simulink model "Rob_Diff_Erno_1R1"  (R2013a)
settings: Solver=ode45  StartTime=0.0  StopTime=inf  RelTol=1e-3
undefined symbols (not defined in the file): Corp1, RoataMare1, Rob_Diff_Erno_1, RootPart
libraries: mblibv1 x17
settings Model: Creator=Claudiu  LastModifiedBy=Claudiu
settings SimMechanicsCC: VisOnUpdateDiagram=on  VisDuringSimulation=on

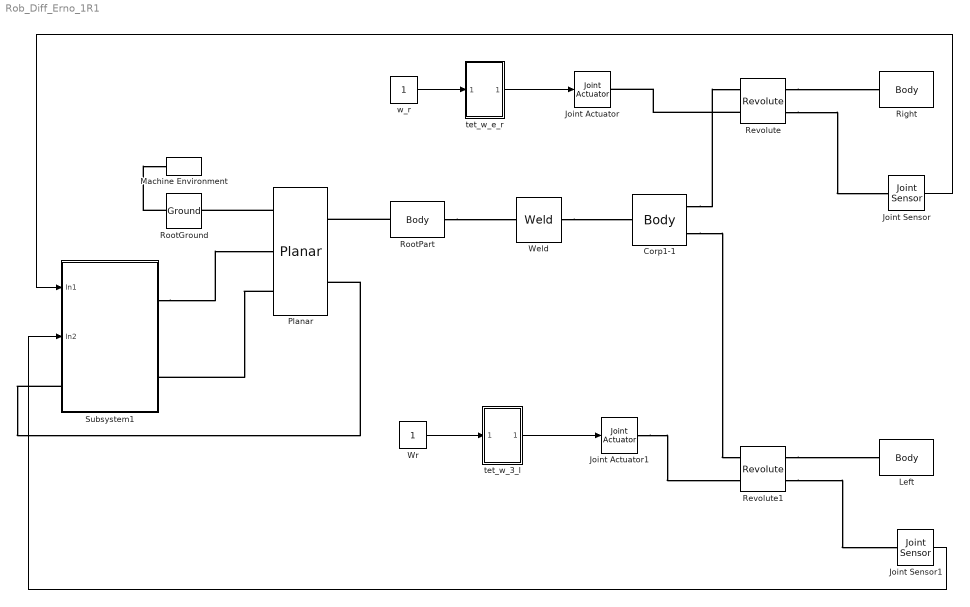
== system Rob_Diff_Erno_1R1 ==
  Corp1-1 : mblibv1/Bodies/Body  LConnTagsString=CS2  RConnTagsString=CS3|CS4  UpdateFromCAD=on  PMImportedID=Corp1-1  DialogClass=MechanicalBodyBlock  Mass=50.6599  MassUnits=kg  InertiaUnits=kg*m^2  Inertia=[1.29318,-0.000149252,5.94621e-08;-0.000149252,0.603177,0.00116217;5.94621e-08,0.00116217,1.81376]  Shape=Cylinder  ShapeDims=[1 1]  ShapeUnits=m  ShapeUse=false  Density=1  DensityUnits=kg/m^3  DensityUse=false  GraphicsMode=GFXFILE  GraphicsFileName=Rob_Diff_Erno_1 - Corp1-1.STL  BodyColorSelMode=COLORPALETTE  BodyColor=[0.894118;0.913725;0.929412]  AttachedToCS=CS1  CG=Right$CG$[-3.54762e-11 0.213212 0.000124454]$WORLD$WORLD$m$[1 0 0;0 1 0;0 0 1]$3x3 Transform$rad$WORLD$false$Corp1-1::CG(AUTOGEN)  WorkingFrames=Right$CS1$[0 0 0]$WORLD$WORLD$m$[1 0 0;0 1 0;0 0 1]$3x3 Transform$rad$WORLD$false$Corp1-1::CS1(AUTOGEN)#Left$CS2$[-3.54762e-11 0.213212 0.000124454]$WORLD$WORLD$m$[1 0 0;0 1 0;0 0 1]$3x3 Transform$rad$WORLD$true$Corp1-1:-:Rob_Diff_Erno_1/RootPart::Corp1-1(AUTOGEN)#Right$CS3$[-0.27 0.253869 0]$WORLD$WORLD$m$[1 0 0;0 1 0;0 0 1]$3x3 Transform$rad$WORLD$true$Corp1-1:-:RoataMare1-1::Corp1-1(AUTOGEN)#Right$CS4$[0.27 0.254678 0]$WORLD$WORLD$m$[1 0 0;0 1 0;0 0 1]$3x3 Transform$rad$WORLD$true$Corp1-1:-:RoataMare1-2::Corp1-1(AUTOGEN)  CGPos=[-3.54762e-11 0.213212 0.000124454]  CGRot=[1 0 0;0 1 0;0 0 1]  CS0Pos=[]  CS0Rot=[]  CS1Pos=[0 0 0]  CS1Rot=[1 0 0;0 1 0;0 0 1]  CS2Pos=[-3.54762e-11 0.213212 0.000124454]  CS2Rot=[1 0 0;0 1 0;0 0 1]  CS3Pos=[-0.27 0.253869 0]  CS3Rot=[1 0 0;0 1 0;0 0 1]  CS4Pos=[0.27 0.254678 0]  CS4Rot=[1 0 0;0 1 0;0 0 1]  CS5Pos=[]  CS5Rot=[]  CS6Pos=[]  CS6Rot=[]  CS7Pos=[]  CS7Rot=[]  CS8Pos=[]  CS8Rot=[]  CS9Pos=[]  CS9Rot=[]  CS10Pos=[]  CS10Rot=[]  CS11Pos=[]  CS11Rot=[]  CS12Pos=[]  CS12Rot=[]  CS13Pos=[]  CS13Rot=[]  CS14Pos=[]  CS14Rot=[]  CS15Pos=[]  CS15Rot=[]  CS16Pos=[]  CS16Rot=[]  CS17Pos=[]  CS17Rot=[]  CS18Pos=[]  CS18Rot=[]  CS19Pos=[]  CS19Rot=[]  CS20Pos=[]  CS20Rot=[]
  Joint Actuator : mblibv1/Sensors &  Actuators/Joint Actuator  UpdateFromCAD=off  PhysicalDomain=Mechanical  PortType=blob  ActuationStyle=Motion  AngleUnits=deg  ArcVelocityUnits=deg/s  ArcAccelerationUnits=deg/s^2  CoordPositionUnits=m  VelocityUnits=m/s  AccelerationUnits=m/s^2  ForceUnits=N  TorqueUnits=N*m  ActiveIO=on  Width=3  DialogClass=MechanicalActuatorBlock  Primitive=R1  ReferenceFrame=Absolute (World)
  Joint Actuator1 : mblibv1/Sensors &  Actuators/Joint Actuator  UpdateFromCAD=off  PhysicalDomain=Mechanical  PortType=blob  ActuationStyle=Motion  AngleUnits=deg  ArcVelocityUnits=deg/s  ArcAccelerationUnits=deg/s^2  CoordPositionUnits=m  VelocityUnits=m/s  AccelerationUnits=m/s^2  ForceUnits=N  TorqueUnits=N*m  ActiveIO=on  Width=3  DialogClass=MechanicalActuatorBlock  Primitive=R1  ReferenceFrame=Absolute (World)
  Joint Sensor : mblibv1/Sensors &  Actuators/Joint Sensor  UpdateFromCAD=off  PhysicalDomain=Mechanical  PortType=blob  Muxed=on  Pose=off  Angle=off  AngleUnits=rad  ArcVelocity=on  ArcVelocityUnits=rad/s  ArcAcceleration=off  ArcAccelerationUnits=deg/s^2  CoordPosition=on  CoordPositionUnits=m  Velocity=off  VelocityUnits=m/s  Acceleration=off  AccelerationUnits=m/s^2  Quaternion=on  QuaternionDT=off  QuaternionDDT=off  QuaternionUnits=off  OutputVector=[1]  ActiveIO=on  Width=1  DialogClass=MechanicalSensorBlock  Primitive=R1  Force=off  ForceUnits=N  Torque=off  TorqueUnits=N*m  ReferenceFrame=Absolute (World)  ReactionSensedSide=Base  ReactionReferenceFrame=Absolute (World)  ReactionForce=off  ReactionForceUnits=N  ReactionMoment=off  ReactionMomentUnits=N*m
  Joint Sensor1 : mblibv1/Sensors &  Actuators/Joint Sensor  UpdateFromCAD=off  PhysicalDomain=Mechanical  PortType=blob  Muxed=on  Pose=off  Angle=off  AngleUnits=rad  ArcVelocity=on  ArcVelocityUnits=rad/s  ArcAcceleration=off  ArcAccelerationUnits=deg/s^2  CoordPosition=on  CoordPositionUnits=m  Velocity=off  VelocityUnits=m/s  Acceleration=off  AccelerationUnits=m/s^2  Quaternion=on  QuaternionDT=off  QuaternionDDT=off  QuaternionUnits=off  OutputVector=[1]  ActiveIO=on  Width=1  DialogClass=MechanicalSensorBlock  Primitive=R1  Force=off  ForceUnits=N  Torque=off  TorqueUnits=N*m  ReferenceFrame=Absolute (World)  ReactionSensedSide=Base  ReactionReferenceFrame=Absolute (World)  ReactionForce=off  ReactionForceUnits=N  ReactionMoment=off  ReactionMomentUnits=N*m
  Left : mblibv1/Bodies/Body  LConnTagsString=CS2  UpdateFromCAD=on  PMImportedID=RoataMare1-2  DialogClass=MechanicalBodyBlock  Mass=3.13776  MassUnits=kg  InertiaUnits=kg*m^2  Inertia=[0.016344,3.64267e-07,-4.71483e-11;3.64267e-07,0.0163435,-1.65655e-11;-4.71483e-11,-1.65655e-11,0.0280968]  Shape=Cylinder  ShapeDims=[1 1]  ShapeUnits=m  ShapeUse=false  Density=1  DensityUnits=kg/m^3  DensityUse=false  GraphicsMode=GFXFILE  GraphicsFileName=Rob_Diff_Erno_1 - RoataMare1-2.STL  BodyColorSelMode=COLORPALETTE  BodyColor=[0.792157;0.819608;0.933333]  AttachedToCS=CS1  CG=Right$CG$[0.22 0.254684 2.07949e-06]$WORLD$WORLD$m$[0 0 -1;0.683357 0.730084 0;0.730084 -0.683357 0]$3x3 Transform$rad$WORLD$false$RoataMare1-2::CG(AUTOGEN)  WorkingFrames=Right$CS1$[0.22 0.254678 0]$WORLD$WORLD$m$[0 0 -1;0.683357 0.730084 0;0.730084 -0.683357 0]$3x3 Transform$rad$WORLD$false$RoataMare1-2::CS1(AUTOGEN)#Left$CS2$[0.27 0.254678 0]$WORLD$WORLD$m$[1 0 0;0 1 0;0 0 1]$3x3 Transform$rad$WORLD$true$Corp1-1:-:RoataMare1-2::RoataMare1-2(AUTOGEN)  CGPos=[0.22 0.254684 2.07949e-06]  CGRot=[0 0 -1;0.683357 0.730084 0;0.730084 -0.683357 0]  CS0Pos=[]  CS0Rot=[]  CS1Pos=[0.22 0.254678 0]  CS1Rot=[0 0 -1;0.683357 0.730084 0;0.730084 -0.683357 0]  CS2Pos=[0.27 0.254678 0]  CS2Rot=[1 0 0;0 1 0;0 0 1]  CS3Pos=[]  CS3Rot=[]  CS4Pos=[]  CS4Rot=[]  CS5Pos=[]  CS5Rot=[]  CS6Pos=[]  CS6Rot=[]  CS7Pos=[]  CS7Rot=[]  CS8Pos=[]  CS8Rot=[]  CS9Pos=[]  CS9Rot=[]  CS10Pos=[]  CS10Rot=[]  CS11Pos=[]  CS11Rot=[]  CS12Pos=[]  CS12Rot=[]  CS13Pos=[]  CS13Rot=[]  CS14Pos=[]  CS14Rot=[]  CS15Pos=[]  CS15Rot=[]  CS16Pos=[]  CS16Rot=[]  CS17Pos=[]  CS17Rot=[]  CS18Pos=[]  CS18Rot=[]  CS19Pos=[]  CS19Rot=[]  CS20Pos=[]  CS20Rot=[]
  Machine Environment : mblibv1/Bodies/Machine Environment  PortType=env  PhysicalDomain=Mechanical  DialogTemplateClass=MECH.MachineEnvironment  SyncWhenCopied=off  Gravity=[0 0 0]  GravityUnits=m/s^2  GravityAsSignal=off  Dimensionality=Auto-detect  AnalysisType=Forward dynamics  LinearAssemblyTolerance=1e-3  LinearAssemblyToleranceUnits=m  AngularAssemblyTolerance=1e-3  AngularAssemblyToleranceUnits=rad  ConstraintSolverType=Stabilizing  ConstraintRelTolerance=1e-4  ConstraintAbsTolerance=1e-4  UseRobustSingularityHandling=off  RedundancyAnalysisToleranceType=Automatically select tolerance  RedundancyAnalysisTolerance=1e-14  StatePerturbationType=Fixed  PerturbationSize=1e-5  VisualizeMachine=on  BodyVisualizationType=Use model default body geometries  BodyColorSelMode=Use model default  DefaultBodyColor=[1 0 0]
  Planar : mblibv1/Joints/Planar  LConnTagsString=__newl0|SA1|SA2  RConnTagsString=__newr0|SA1  UpdateFromCAD=off  NumSAPorts=3  CutJoint=off  MarkAsCut=off  Primitives=prismatic_prismatic  PrimitiveProps=P1$World$[1 0 0]$prismatic#P2$World$[0 1 0]$prismatic#R1$World$[0 0 1]$revolute  DialogClass=JointBlock  P1Axis=[1 0 0]  P2Axis=[0 1 0]  R1Axis=[0 0 1]
  Revolute : mblibv1/Joints/Revolute  LConnTagsString=__newl0|SA1  RConnTagsString=__newr0|SA1  UpdateFromCAD=on  PMImportedID=Corp1-1:-:RoataMare1-1  NumSAPorts=2  CutJoint=off  MarkAsCut=off  Primitives=prismatic  PrimitiveProps=R1$World$[1,0,0]$revolute  DialogClass=JointBlock  R1Axis=[1,0,0]
  Revolute1 : mblibv1/Joints/Revolute  LConnTagsString=__newl0|SA1  RConnTagsString=__newr0|SA1  UpdateFromCAD=on  PMImportedID=Corp1-1:-:RoataMare1-2  NumSAPorts=2  CutJoint=off  MarkAsCut=off  Primitives=prismatic  PrimitiveProps=R1$World$[-1,0,0]$revolute  DialogClass=JointBlock  R1Axis=[-1,0,0]
  Right : mblibv1/Bodies/Body  LConnTagsString=CS2  UpdateFromCAD=on  PMImportedID=RoataMare1-1  DialogClass=MechanicalBodyBlock  Mass=3.13776  MassUnits=kg  InertiaUnits=kg*m^2  Inertia=[0.016344,3.64267e-07,-4.71483e-11;3.64267e-07,0.0163435,-1.65655e-11;-4.71483e-11,-1.65655e-11,0.0280968]  Shape=Cylinder  ShapeDims=[1 1]  ShapeUnits=m  ShapeUse=false  Density=1  DensityUnits=kg/m^3  DensityUse=false  GraphicsMode=GFXFILE  GraphicsFileName=Rob_Diff_Erno_1 - RoataMare1-1.STL  BodyColorSelMode=COLORPALETTE  BodyColor=[0.792157;0.819608;0.933333]  AttachedToCS=CS1  CG=Right$CG$[-0.22 0.253871 -6.67283e-06]$WORLD$WORLD$m$[0 0 1;-0.325894 0.945406 0;-0.945406 -0.325894 0]$3x3 Transform$rad$WORLD$false$RoataMare1-1::CG(AUTOGEN)  WorkingFrames=Right$CS1$[-0.22 0.253869 0]$WORLD$WORLD$m$[0 0 1;-0.325894 0.945406 0;-0.945406 -0.325894 0]$3x3 Transform$rad$WORLD$false$RoataMare1-1::CS1(AUTOGEN)#Left$CS2$[-0.27 0.253869 0]$WORLD$WORLD$m$[1 0 0;0 1 0;0 0 1]$3x3 Transform$rad$WORLD$true$Corp1-1:-:RoataMare1-1::RoataMare1-1(AUTOGEN)  CGPos=[-0.22 0.253871 -6.67283e-06]  CGRot=[0 0 1;-0.325894 0.945406 0;-0.945406 -0.325894 0]  CS0Pos=[]  CS0Rot=[]  CS1Pos=[-0.22 0.253869 0]  CS1Rot=[0 0 1;-0.325894 0.945406 0;-0.945406 -0.325894 0]  CS2Pos=[-0.27 0.253869 0]  CS2Rot=[1 0 0;0 1 0;0 0 1]  CS3Pos=[]  CS3Rot=[]  CS4Pos=[]  CS4Rot=[]  CS5Pos=[]  CS5Rot=[]  CS6Pos=[]  CS6Rot=[]  CS7Pos=[]  CS7Rot=[]  CS8Pos=[]  CS8Rot=[]  CS9Pos=[]  CS9Rot=[]  CS10Pos=[]  CS10Rot=[]  CS11Pos=[]  CS11Rot=[]  CS12Pos=[]  CS12Rot=[]  CS13Pos=[]  CS13Rot=[]  CS14Pos=[]  CS14Rot=[]  CS15Pos=[]  CS15Rot=[]  CS16Pos=[]  CS16Rot=[]  CS17Pos=[]  CS17Rot=[]  CS18Pos=[]  CS18Rot=[]  CS19Pos=[]  CS19Rot=[]  CS20Pos=[]  CS20Rot=[]
  RootGround : mblibv1/Bodies/Ground  UpdateFromCAD=on  PMImportedID=RootGround  LeftPortType=env  RightPortType=workingframe  PhysicalDomain=Mechanical  DialogClass=GroundBlock  CoordPosition=[-3.1566e-11,0.217738,0.000110483]  CoordPositionUnits=m  StateVectorMgrId=0  MachineId=[1 0]  ShowEnvPort=on
  RootPart : mblibv1/Bodies/Body  LConnTagsString=CS3  RConnTagsString=CS2  UpdateFromCAD=on  PMImportedID=Rob_Diff_Erno_1/RootPart  DialogClass=MechanicalBodyBlock  Mass=0  MassUnits=kg  InertiaUnits=kg*m^2  Inertia=[0,0,0;0,0,0;0,0,0]  Shape=Cylinder  ShapeDims=[1 1]  ShapeUnits=m  ShapeUse=false  Density=1  DensityUnits=kg/m^3  DensityUse=false  GraphicsMode=MACHINE_DEFAULT  BodyColorSelMode=MACHINE_DEFAULT  BodyColor=[1;0;0]  AttachedToCS=CS1  CG=Right$CG$[-3.1566e-11 0.217738 0.000110483]$WORLD$WORLD$m$[1 0 0;0 1 0;0 0 1]$3x3 Transform$rad$WORLD$false$Rob_Diff_Erno_1/RootPart::CG(AUTOGEN)  WorkingFrames=Right$CS1$[0 0 0]$WORLD$WORLD$m$[1 0 0;0 1 0;0 0 1]$3x3 Transform$rad$WORLD$false$Rob_Diff_Erno_1/RootPart::CS1(AUTOGEN)#Right$CS2$[-3.54762e-11 0.213212 0.000124454]$WORLD$WORLD$m$[1 0 0;0 1 0;0 0 1]$3x3 Transform$rad$WORLD$true$Corp1-1:-:Rob_Diff_Erno_1/RootPart::Rob_Diff_Erno_1/RootPart(AUTOGEN)#Left$CS3$[-3.1566e-11 0.217738 0.000110483]$WORLD$WORLD$m$[1 0 0;0 1 0;0 0 1]$3x3 Transform$rad$WORLD$true$Rob_Diff_Erno_1/RootPart:-:RootGround::Rob_Diff_Erno_1/RootPart(AUTOGEN)  CGPos=[-3.1566e-11 0.217738 0.000110483]  CGRot=[1 0 0;0 1 0;0 0 1]  CS0Pos=[]  CS0Rot=[]  CS1Pos=[0 0 0]  CS1Rot=[1 0 0;0 1 0;0 0 1]  CS2Pos=[-3.54762e-11 0.213212 0.000124454]  CS2Rot=[1 0 0;0 1 0;0 0 1]  CS3Pos=[-3.1566e-11 0.217738 0.000110483]  CS3Rot=[1 0 0;0 1 0;0 0 1]  CS4Pos=[]  CS4Rot=[]  CS5Pos=[]  CS5Rot=[]  CS6Pos=[]  CS6Rot=[]  CS7Pos=[]  CS7Rot=[]  CS8Pos=[]  CS8Rot=[]  CS9Pos=[]  CS9Rot=[]  CS10Pos=[]  CS10Rot=[]  CS11Pos=[]  CS11Rot=[]  CS12Pos=[]  CS12Rot=[]  CS13Pos=[]  CS13Rot=[]  CS14Pos=[]  CS14Rot=[]  CS15Pos=[]  CS15Rot=[]  CS16Pos=[]  CS16Rot=[]  CS17Pos=[]  CS17Rot=[]  CS18Pos=[]  CS18Rot=[]  CS19Pos=[]  CS19Rot=[]  CS20Pos=[]  CS20Rot=[]
  Subsystem1 : Subsystem
  Weld : mblibv1/Joints/Weld  LConnTagsString=__newl0  RConnTagsString=__newr0  UpdateFromCAD=on  PMImportedID=Corp1-1:-:Rob_Diff_Erno_1/RootPart  NumSAPorts=0  CutJoint=off  MarkAsCut=off  Primitives=weld  PrimitiveProps=W$WORLD$[0.57735,0.57735,0.57735]$weld  DialogClass=JointBlock  WAxis=[0.57735,0.57735,0.57735]
  Wr : Constant
  tet_w_3_l : Subsystem
  tet_w_e_r : Subsystem
  w_r : Constant
  wires:
  w_r/1 -> tet_w_e_r/1(In1)
  tet_w_e_r/1(Out1) -> Joint Actuator/1
  Wr/1 -> tet_w_3_l/1(In1)
  tet_w_3_l/1(Out1) -> Joint Actuator1/1
  Joint Sensor/1 -> Subsystem1/1(In1)
  Joint Sensor1/1 -> Subsystem1/2(In2)
  connections:
  RootPart/RConn1 -- Weld/LConn1
  Weld/RConn1 -- Corp1-1/LConn1
  Corp1-1/RConn1 -- Revolute/LConn1
  Revolute/RConn1 -- Right/LConn1
  Corp1-1/RConn2 -- Revolute1/LConn1
  Revolute1/RConn1 -- Left/LConn1
  Planar/LConn1 -- RootGround/RConn1
  RootPart/LConn1 -- Planar/RConn1
  RootGround/LConn1 -- Machine Environment/RConn1
  Revolute/LConn2 -- Joint Actuator/RConn1
  Joint Actuator1/RConn1 -- Revolute1/LConn2
  Revolute/RConn2 -- Joint Sensor/LConn1
  Revolute1/RConn2 -- Joint Sensor1/LConn1
  Subsystem1/RConn1 -- Planar/LConn2
  Subsystem1/LConn1 -- Planar/RConn2
  Planar/LConn3 -- Subsystem1/RConn2

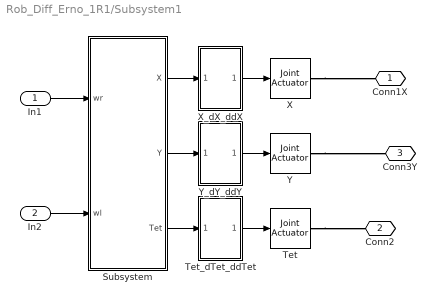
== system Rob_Diff_Erno_1R1/Subsystem1 ==
  In1 : Inport
  In2 : Inport  Port=2
  Subsystem : Subsystem
  Tet : mblibv1/Sensors &  Actuators/Joint Actuator  UpdateFromCAD=off  PhysicalDomain=Mechanical  PortType=blob  ActuationStyle=Motion  AngleUnits=deg  ArcVelocityUnits=deg/s  ArcAccelerationUnits=deg/s^2  CoordPositionUnits=m  VelocityUnits=m/s  AccelerationUnits=m/s^2  ForceUnits=N  TorqueUnits=N*m  ActiveIO=on  Width=3  DialogClass=MechanicalActuatorBlock  Primitive=R1  ReferenceFrame=Absolute (World)
  Tet_dTet_ddTet : Subsystem
  X : mblibv1/Sensors &  Actuators/Joint Actuator  UpdateFromCAD=off  PhysicalDomain=Mechanical  PortType=blob  ActuationStyle=Motion  AngleUnits=deg  ArcVelocityUnits=deg/s  ArcAccelerationUnits=deg/s^2  CoordPositionUnits=m  VelocityUnits=m/s  AccelerationUnits=m/s^2  ForceUnits=N  TorqueUnits=N*m  ActiveIO=on  Width=3  DialogClass=MechanicalActuatorBlock  Primitive=P1  ReferenceFrame=Absolute (World)
  X_dX_ddX : Subsystem
  Y : mblibv1/Sensors &  Actuators/Joint Actuator  UpdateFromCAD=off  PhysicalDomain=Mechanical  PortType=blob  ActuationStyle=Motion  AngleUnits=deg  ArcVelocityUnits=deg/s  ArcAccelerationUnits=deg/s^2  CoordPositionUnits=m  VelocityUnits=m/s  AccelerationUnits=m/s^2  ForceUnits=N  TorqueUnits=N*m  ActiveIO=on  Width=3  DialogClass=MechanicalActuatorBlock  Primitive=P2  ReferenceFrame=Absolute (World)
  Y_dY_ddY : Subsystem
  Conn1X : PMIOPort  Port=1  Side=Right
  Conn2 : PMIOPort  Port=2  Side=Left
  Conn3Y : PMIOPort  Port=3  Side=Right
  wires:
  Subsystem/1(X) -> X_dX_ddX/1(In3)
  Subsystem/3(Tet) -> Tet_dTet_ddTet/1(In3)
  Subsystem/2(Y) -> Y_dY_ddY/1(In3)
  In1/1 -> Subsystem/1(wr)
  In2/1 -> Subsystem/2(wl)
  X_dX_ddX/1(Out1) -> X/1
  Y_dY_ddY/1(Out1) -> Y/1
  Tet_dTet_ddTet/1(Out1) -> Tet/1
  connections:
  Tet/RConn1 -- Conn2/RConn1
  X/RConn1 -- Conn1X/RConn1
  Y/RConn1 -- Conn3Y/RConn1

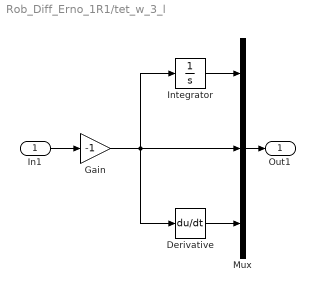
== system Rob_Diff_Erno_1R1/tet_w_3_l ==
  In1 : Inport
  Derivative : Derivative
  Gain : Gain  Gain=-1
  Integrator : Integrator
  Mux : Mux  Inputs=3
  Out1 : Outport
  wires:
  Mux/1 -> Out1/1
  Derivative/1 -> Mux/3
  Integrator/1 -> Mux/1
  In1/1 -> Gain/1
  Gain/1 -> Integrator/1, Mux/2, Derivative/1

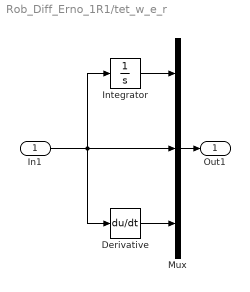
== system Rob_Diff_Erno_1R1/tet_w_e_r ==
  In1 : Inport
  Derivative : Derivative
  Integrator : Integrator
  Mux : Mux  Inputs=3
  Out1 : Outport
  wires:
  In1/1 -> Integrator/1, Derivative/1, Mux/2
  Integrator/1 -> Mux/1
  Derivative/1 -> Mux/3
  Mux/1 -> Out1/1

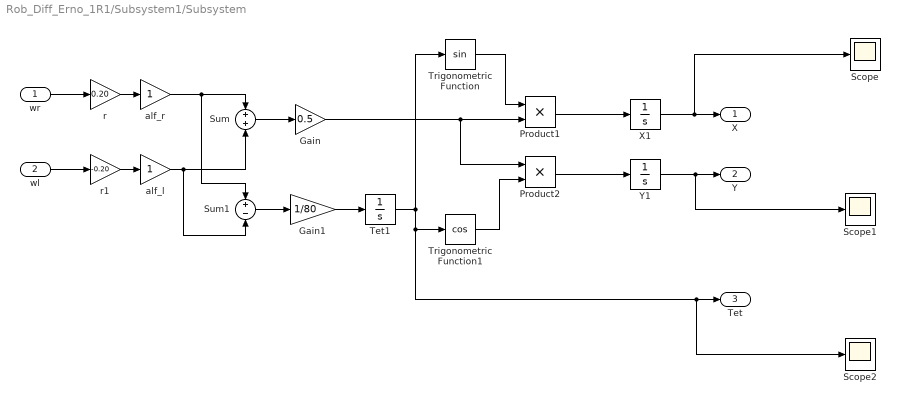
== system Rob_Diff_Erno_1R1/Subsystem1/Subsystem ==
  wr : Inport
  wl : Inport  Port=2
  Gain : Gain  Gain=0.5
  Gain1 : Gain  Gain=1/80
  Product1 : Product
  Product2 : Product
  Scope : Scope
  Scope1 : Scope
  Scope2 : Scope
      settings: SaveName=ScopeData2
  Sum : Sum
  Sum1 : Sum  Inputs=+-
  Tet1 : Integrator
  Trigonometric Function : Trigonometry
  Trigonometric Function1 : Trigonometry  Operator=cos
  X1 : Integrator
  Y1 : Integrator
  alf_l : Gain
  alf_r : Gain
  r : Gain  Gain=0.20
  r1 : Gain  Gain=-0.20
  X : Outport
  Y : Outport  Port=2
  Tet : Outport  Port=3
  wires:
  alf_l/1 -> Sum/2, Sum1/2
  alf_r/1 -> Sum1/1, Sum/1
  r1/1 -> alf_l/1
  r/1 -> alf_r/1
  Gain1/1 -> Tet1/1
  Gain/1 -> Product2/1, Product1/2
  Sum1/1 -> Gain1/1
  wl/1 -> r1/1
  wr/1 -> r/1
  Product2/1 -> Y1/1
  Product1/1 -> X1/1
  Sum/1 -> Gain/1
  Trigonometric Function1/1 -> Product2/2
  Trigonometric Function/1 -> Product1/1
  Tet1/1 -> Trigonometric Function/1, Scope2/1, Tet/1, Trigonometric Function1/1
  X1/1 -> Scope/1, X/1
  Y1/1 -> Scope1/1, Y/1

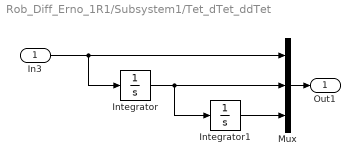
== system Rob_Diff_Erno_1R1/Subsystem1/Tet_dTet_ddTet ==
  In3 : Inport
  Integrator : Integrator
  Integrator1 : Integrator
  Mux : Mux  Inputs=3
  Out1 : Outport
  wires:
  In3/1 -> Integrator/1, Mux/1
  Integrator/1 -> Integrator1/1, Mux/2
  Mux/1 -> Out1/1
  Integrator1/1 -> Mux/3

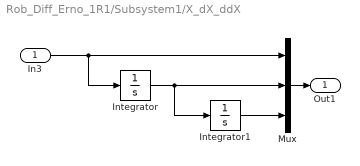
== system Rob_Diff_Erno_1R1/Subsystem1/X_dX_ddX ==
  In3 : Inport
  Integrator : Integrator
  Integrator1 : Integrator
  Mux : Mux  Inputs=3
  Out1 : Outport
  wires:
  In3/1 -> Integrator/1, Mux/1
  Integrator/1 -> Integrator1/1, Mux/2
  Mux/1 -> Out1/1
  Integrator1/1 -> Mux/3

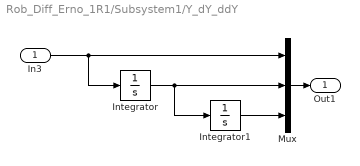
== system Rob_Diff_Erno_1R1/Subsystem1/Y_dY_ddY ==
  In3 : Inport
  Integrator : Integrator
  Integrator1 : Integrator
  Mux : Mux  Inputs=3
  Out1 : Outport
  wires:
  Integrator1/1 -> Mux/3
  Mux/1 -> Out1/1
  Integrator/1 -> Mux/2, Integrator1/1
  In3/1 -> Mux/1, Integrator/1
